simulink model "vr_octavia"  (Simulink 7.5)
settings: Solver=ode45  StartTime=0.0  StopTime=111.56  RelTol=1e-3
PostLoadFcn:
  | load octavia_testlap
libraries: vrlib x26, simulink x1
Description:
  | Vehicle Dynamics Visualization
  | 
  | The vr_octavia example shows the benefits of visualization of complex dynamic model
  | in the virtual reality environment. It also demonstrates Simulink(R) 3D Animation(TM)
  | 3D off-line animation recording functionality.
  | 
  | The pre-computed simulation data, representing one lap of a vehicle on a testing circuit,
  | is converted from dynamic model signal structure into the form that can be sent
  | to the virtual reality scene. This conversion includes splitting the combined signals
  | into signals governing individual VRML objects properties and coordinate systems
  | transformations. The data is then sent to the virtual reality scene using
  | VR Sink block with sample rate 25 Hz.
  | 
  | The dynamic model provides not only signals that influence visual properties of objects
  | (positions and rotations), but also forces and other similar quantities, that can be
  | visualized as well. In this example, wheel forces are visualized using VRML triads
  | scaled dynamically according to current force values. Force triads can be switched off
  | by the Forces Visibility Switch.
  | 
  | When working with virtual reality models, there is a common requirement to track
  | certain moving objects with the camera. Usually, the direction from the camera
  | to the object is easily available (both positions are known, so direction from
  | the camera to the object is defined as the difference between the two positions).
  | Because in VRML the viewpoint orientation is defined in the form of 4-element [axis angle]
  | VRML rotation, camera direction must be converted into this format before sending
  | to virtual scene. Simulink 3D Animation provides the Viewpoint Direction to VRML Orientation
  | block to perform this conversion. In this example, switch to the "Simulink Controlled Viewpoint"
  | in the viewer to see the camera tracking effect.
  | 
  | Simulink 3D Animation allows two methods of recording animation files - 2D animation (AVI files)
  | and 3D animation (VRML files). Here we describe how a 3D VRML animation file can be
  | created and further used. In the internal viewer Recording menu select the
  | Capture and Recording Parameters... option.
  | 
  | In the Capture and Recording Parameters dialog, select the Record to VRML checkbox.
  | Leave the File: editbox at its default value. Select the Scheduled Recording mode
  | and specify the time period for which you want to record the offline animation time.
  | Here we record the animation during the entire simulation time defined for this model,
  | you may select any time interval between the Simulink model Start time and Stop time.
  | For details on recording parameters please refer to the product documentation.
  | 
  | Once you define these animation recording parameters, animation file is created
  | automatically when you start the simulation. Unlike with creating the 2D animation files,
  | the internal viewer figure can be minimized during simulation, which significantly speeds up
  | the simulation. At the end of simulation run, the created VRML animation file
  | octavia_scene_anim_1.wrl remains in the working directory for later use.
  | 
  | If you distribute animation files, make sure to also distribute all the inlined object and texture
  | files referenced in the original VRML world file.
  | 
  | In the case of this demonstration example, the following files must be distributed together
  | with the resulting animation file octavia_scene_anim_1.wrl :
  | 
  |     * octavia_body.wrl
  |     * octavia_road.wrl
  |     * triad.wrl
  |     * /texture/octavia_*.jpg
  | 
  | As the VRML animation file is created by default into the current working directory,
  | and not the Simulink 3D Animation demos directory, you will need to copy all these
  | files to the current working directory to view the off-line animation file correctly.
  | 
  | Viewing VRML off-line animation file:
  | 
  | Let's assume that you want to view the octavia_scene_anim_1.wrl file that is in your
  | current working directory. You can play and inspect this animated file with comfort
  | using the VR Animation Player tool:
  | 
  |     vrplay('octavia_scene_anim_1.wrl');
  | 
  | You can view the resulting VRML animation file also using Orbisnap, blaxxun Contact
  | or any other generally available VRML97 viewer, or using Simulink 3D Animation
  | Internal Viewer. When using the internal viewer, it is necessary to set the virtual world
  | TimeSource property to freerun to be able to see the animation. Issue the following
  | commands at the MATLAB(R) command window:
  | 
  |     w=vrview('octavia_scene_anim_1.wrl');
  |     set(w, 'TimeSource', 'freerun');
  | 
  | A VRML animation file based on this example is pre-recorded in the /vrdemos directory
  | under the following name:
  | 
  |     octavia_scene_anim.wrl
  | 
  | Acknowledgements:
  | 
  | Skoda Octavia model copyright Skoda Auto, courtesy of Ismar VR, Czech Republic.
  | Road geometry and simulation data generated using veDYNA by TESIS DYNAware, Germany.
settings Model: Creator=Sehnal  LastModifiedBy=Danek  ExtModeArmWhenConnect=off  BufferReuse=off
settings DataIOCC: SignalLoggingName=sigsOut
settings OptimizationCC: BooleanDataType=off  InlineInvariantSignals=on  OptimizeBlockIOStorage=off  BufferReuse=off  ExpressionFolding=off  LocalBlockOutputs=off  InitFltsAndDblsToZero=on
settings DebuggingCC: CheckExecutionContextPreStartOutputMsg=on  CheckExecutionContextRuntimeOutputMsg=on  SignalResolutionControl=TryResolveAllWithWarning  SolverPrmCheckMsg=none  MultiTaskDSMMsg=warning  MultiTaskCondExecSysMsg=none  StrictBusMsg=None
settings RTWCC: RetainRTWFile=on  ProcessScript=grt_make_rtw_hook  IncludeERTFirstTime=on
settings GRTTargetCC: TargetFcnLib=ansi_tfl_tmw.mat

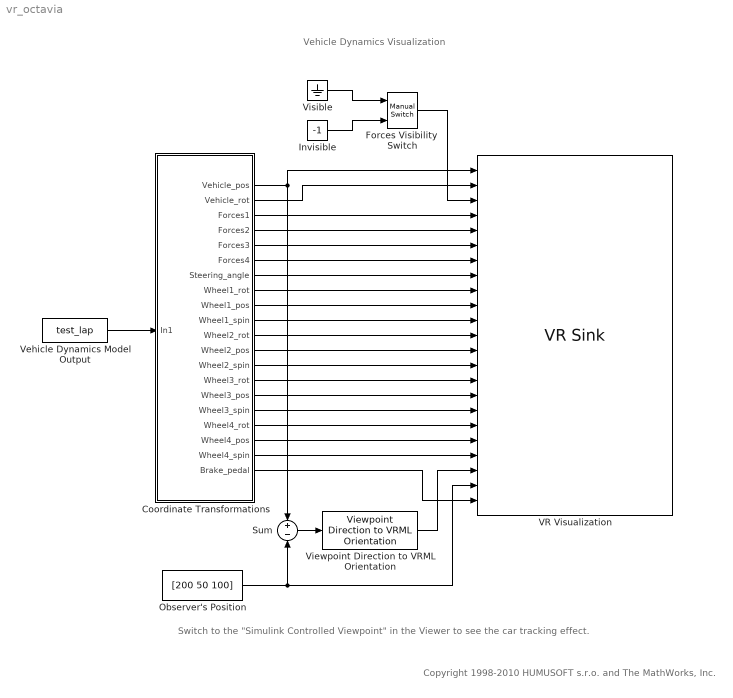
== system vr_octavia ==
  note: Vehicle Dynamics Visualization
  note: Switch to the "Simulink Controlled Viewpoint"
      | in the Viewer to see the car tracking effect.
  note: Copyright 1998-2010 HUMUSOFT s.r.o. and The MathWorks, Inc.
  Coordinate Transformations : Subsystem
  Forces Visibility  Switch : simulink/Signal Routing/Manual Switch  SystemSampleTime=-1  sw=1  action=0  varsize=off
  Invisible : Constant  Value=-1  OutDataType=sfix(16)  OutScaling=2^0
  Observer's Position : Constant  Value=[200 50 100]  OutDataType=sfix(16)  OutScaling=2^0
  Sum : Sum  Inputs=+-  OutDataType=sfix(16)  OutScaling=2^0
  VR Visualization : vrlib/VR Sink  InstantiateOnLoad=on  SampleTime=0.04  ViewEnable=on  RemoteChange=off  RemoteView=on  FieldsWritten=Vehicle_pos_Car1.translation.3.1.double#Vehicle_rot_Car1.rotation.4.1.double#Forces_visible_Car1.whichChoice.1.1.double#Force1_Car1.scale.3.1.double#Force2_Car1.scale.3.1.double#Force3_Car1.scale.3.1.double#Force4_Car1.scale.3.1.double#SteeringWheelAngle1_Car1.rotation.4.1.double#WheelFL_Car1.rotation.4.1.double#WheelFL_Car1.translation.3.1.double#WheelSpinFL_Car1.rotation.4.1.double#WheelFR_Car1.rotation.4.1.double#WheelFR_Car1.translation.3.1.double#WheelSpinFR_Car1.rotation.4.1.double#WheelRL_Car1.rotation.4.1.double#WheelRL_Car1.translation.3.1.double#WheelSpinRL_Car1.rotation.4.1.double#WheelRR_Car1.rotation.4.1.double#WheelRR_Car1.translation.3.1.double#WheelSpinRR_Car1.rotation.4.1.double#FlyingCamera.orientation.4.1.double#FlyingCamera.position.3.1.double#Brake_Switch_Car1.whichChoice.1.1.double  WorldFileName=octavia_scene.wrl  WorldDescription=Vehicle Dynamics Visualization - Skoda Octavia  AutoView=on  VideoDimensions=[]  FigureProperties="{'Position', 'Name', 'Viewpoint', 'CameraBound', 'CameraDirection', 'CameraPosition', 'CameraUpVector', 'ZoomFactor', 'Antialiasing', 'Headlight', 'Lighting', 'NavPanel', 'StatusBar', 'ToolBar', 'Textures', 'Transparency', 'Wireframe', 'NavZones', 'NavMode', 'NavSpeed', 'Record2DCompressMethod', 'Record2DCompressQuality', 'Record2D', 'Record2DFileName', 'Record2DFPS'; [1.3000000000000000e+001  7.7000000000000000e+001  5.7600000000000000e+002  3.8000000000000000e+002], 'Vehicle Dynamics Visualization - Skoda Octavia', 'Car - View from Right Above Ahead', 'on', [0.0000000000000000e+000  0.0000000000000000e+000 -1.0000000000000000e+000], [0.0000000000000000e+000  0.0000000000000000e+000  0.0000000000000000e+000], [0.0000000000000000e+000  1.0000000000000000e+000  0.0000000000000000e+000], [1.0000000000000000e+000], 'off', 'off', 'on', 'halfbar', 'off', 'on', 'on', 'on', 'off', 'off', 'walk', 'normal', 'auto', [7.5000000000000000e+001], 'off', '%f_anim_%n.avi', [1.5000000000000000e+001]}"
  Vehicle Dynamics Model Output : FromWorkspace  VariableName=test_lap  SampleTime=0.04  OutputAfterFinalValue=Holding final value
  Viewpoint Direction to VRML Orientation : vrlib/Utilities/Viewpoint Direction to VRML Orientation  SystemSampleTime=-1
  Visible : Ground
  wires:
  Visible/1 -> Forces Visibility  Switch/1
  Invisible/1 -> Forces Visibility  Switch/2
  Vehicle Dynamics Model Output/1 -> Coordinate Transformations/1(In1)
  Coordinate Transformations/1(Vehicle_pos) -> VR Visualization/1, Sum/1
  Coordinate Transformations/2(Vehicle_rot) -> VR Visualization/2
  Forces Visibility  Switch/1 -> VR Visualization/3
  Coordinate Transformations/3(Forces1) -> VR Visualization/4
  Coordinate Transformations/4(Forces2) -> VR Visualization/5
  Coordinate Transformations/5(Forces3) -> VR Visualization/6
  Coordinate Transformations/6(Forces4) -> VR Visualization/7
  Coordinate Transformations/7(Steering_angle) -> VR Visualization/8
  Coordinate Transformations/8(Wheel1_rot) -> VR Visualization/9
  Coordinate Transformations/9(Wheel1_pos) -> VR Visualization/10
  Coordinate Transformations/10(Wheel1_spin) -> VR Visualization/11
  Coordinate Transformations/11(Wheel2_rot) -> VR Visualization/12
  Coordinate Transformations/12(Wheel2_pos) -> VR Visualization/13
  Coordinate Transformations/13(Wheel2_spin) -> VR Visualization/14
  Coordinate Transformations/14(Wheel3_rot) -> VR Visualization/15
  Coordinate Transformations/15(Wheel3_pos) -> VR Visualization/16
  Coordinate Transformations/16(Wheel3_spin) -> VR Visualization/17
  Coordinate Transformations/17(Wheel4_rot) -> VR Visualization/18
  Coordinate Transformations/18(Wheel4_pos) -> VR Visualization/19
  Coordinate Transformations/19(Wheel4_spin) -> VR Visualization/20
  Coordinate Transformations/20(Brake_pedal) -> VR Visualization/23
  Sum/1 -> Viewpoint Direction to VRML Orientation/1
  Viewpoint Direction to VRML Orientation/1 -> VR Visualization/21
  Observer's Position/1 -> VR Visualization/22, Sum/2

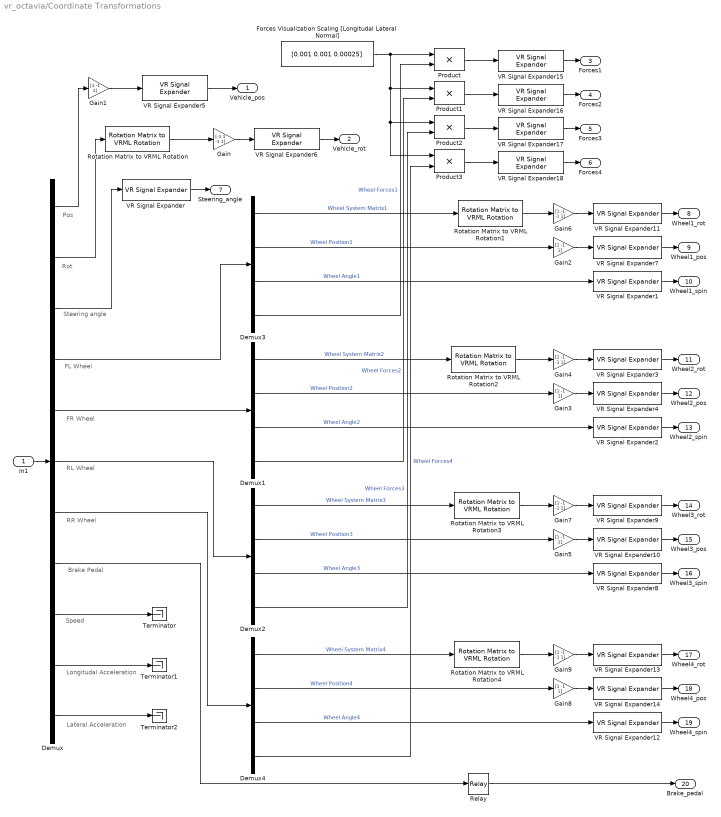
== system vr_octavia/Coordinate Transformations ==
  note: Steering angle
  note: FL Wheel
  note: FR Wheel
  note: RL Wheel
  note: RR Wheel
  note: Brake Pedal
  note: Pos
  note: Rot
  note: Speed
  note: Longitudal Acceleration
  note: Lateral Acceleration
  In1 : Inport  OutDataType=sfix(16)  OutScaling=2^0
  Demux : Demux  Outputs=[3,9,1,16,16,16,16,1,1,1,1]
  Demux{1..4} (4 alike) : Demux  Outputs=[9,3,1,3]
  Forces Visualization Scaling [Longitudal Lateral Normal] : Constant  Value=[0.001 0.001 0.00025]  OutDataType=sfix(16)  OutScaling=2^0
  Gain : Gain  Gain=[-1 1 -1 1]  ParameterDataType=sfix(16)  ParameterScaling=2^0  OutDataType=sfix(16)  OutScaling=2^0  SaturateOnIntegerOverflow=on  OutDataTypeStr=Inherit: Same as input  ParamDataTypeStr=Inherit: Same as input
  Gain{1..3,5,8} (5 alike) : Gain  Gain=[1 -1 1]  ParameterDataType=sfix(16)  ParameterScaling=2^0  OutDataType=sfix(16)  OutScaling=2^0  SaturateOnIntegerOverflow=on  OutDataTypeStr=Inherit: Same as input  ParamDataTypeStr=Inherit: Same as input
  Gain{4,6..7,9} (4 alike) : Gain  Gain=[1 -1 -1 1]  ParameterDataType=sfix(16)  ParameterScaling=2^0  OutDataType=sfix(16)  OutScaling=2^0  SaturateOnIntegerOverflow=on  OutDataTypeStr=Inherit: Same as input  ParamDataTypeStr=Inherit: Same as input
  Product{,1..3} (4 alike) : Product  OutDataType=sfix(16)  OutScaling=2^0  SaturateOnIntegerOverflow=on  OutDataTypeStr=Inherit: Same as first input
  Relay : Relay  OutDataType=sfix(16)  OutScaling=2^0
  Rotation Matrix to VRML Rotation{,1..4} (5 alike) : vrlib/Utilities/Rotation Matrix to VRML Rotation  SystemSampleTime=-1  maxzero=1e-12
  Terminator : Terminator
  Terminator1 : Terminator
  Terminator2 : Terminator
  VR Signal Expander{,1..2,8,12} (5 alike) : vrlib/VR Signal Expander  SystemSampleTime=-1  outwidth=4  outidx=[4]
  VR Signal Expander{4,7,10,14} (4 alike) : vrlib/VR Signal Expander  SystemSampleTime=-1  outwidth=3  outidx=[1 3 2 ]
  VR Signal Expander{3,6,9,11,13} (5 alike) : vrlib/VR Signal Expander  SystemSampleTime=-1  outwidth=4  outidx=[1 3 2 4]
  VR Signal Expander{5,15..18} (5 alike) : vrlib/VR Signal Expander  SystemSampleTime=-1  outwidth=3  outidx=[1 3 2]
  Vehicle_pos : Outport  OutDataType=sfix(16)  OutScaling=2^0
  Vehicle_rot : Outport  Port=2  OutDataType=sfix(16)  OutScaling=2^0
  Forces1 : Outport  Port=3  OutDataType=sfix(16)  OutScaling=2^0
  Forces2 : Outport  Port=4  OutDataType=sfix(16)  OutScaling=2^0
  Forces3 : Outport  Port=5  OutDataType=sfix(16)  OutScaling=2^0
  Forces4 : Outport  Port=6  OutDataType=sfix(16)  OutScaling=2^0
  Steering_angle : Outport  Port=7  OutDataType=sfix(16)  OutScaling=2^0
  Wheel1_rot : Outport  Port=8  OutDataType=sfix(16)  OutScaling=2^0
  Wheel1_pos : Outport  Port=9  OutDataType=sfix(16)  OutScaling=2^0
  Wheel1_spin : Outport  Port=10  OutDataType=sfix(16)  OutScaling=2^0
  Wheel2_rot : Outport  Port=11  OutDataType=sfix(16)  OutScaling=2^0
  Wheel2_pos : Outport  Port=12  OutDataType=sfix(16)  OutScaling=2^0
  Wheel2_spin : Outport  Port=13  OutDataType=sfix(16)  OutScaling=2^0
  Wheel3_rot : Outport  Port=14  OutDataType=sfix(16)  OutScaling=2^0
  Wheel3_pos : Outport  Port=15  OutDataType=sfix(16)  OutScaling=2^0
  Wheel3_spin : Outport  Port=16  OutDataType=sfix(16)  OutScaling=2^0
  Wheel4_rot : Outport  Port=17  OutDataType=sfix(16)  OutScaling=2^0
  Wheel4_pos : Outport  Port=18  OutDataType=sfix(16)  OutScaling=2^0
  Wheel4_spin : Outport  Port=19  OutDataType=sfix(16)  OutScaling=2^0
  Brake_pedal : Outport  Port=20  OutDataType=sfix(16)  OutScaling=2^0
  wires:
  Gain1/1 -> VR Signal Expander5/1
  Rotation Matrix to VRML Rotation/1 -> Gain/1
  Gain/1 -> VR Signal Expander6/1
  Gain6/1 -> VR Signal Expander11/1
  Gain2/1 -> VR Signal Expander7/1
  Demux3/1 -> Rotation Matrix to VRML Rotation1/1  "Wheel System Matrix1"
  Demux3/2 -> Gain2/1  "Wheel Position1"
  Demux3/3 -> VR Signal Expander1/1  "Wheel Angle1"
  Gain4/1 -> VR Signal Expander3/1
  Rotation Matrix to VRML Rotation2/1 -> Gain4/1
  Gain3/1 -> VR Signal Expander4/1
  Demux1/1 -> Rotation Matrix to VRML Rotation2/1  "Wheel System Matrix2"
  Demux1/2 -> Gain3/1  "Wheel Position2"
  Demux1/3 -> VR Signal Expander2/1  "Wheel Angle2"
  Gain7/1 -> VR Signal Expander9/1
  Rotation Matrix to VRML Rotation3/1 -> Gain7/1
  Demux2/4 -> Product2/2  "Wheel Forces3"
  Gain5/1 -> VR Signal Expander10/1
  Demux2/1 -> Rotation Matrix to VRML Rotation3/1  "Wheel System Matrix3"
  Demux2/2 -> Gain5/1  "Wheel Position3"
  Demux2/3 -> VR Signal Expander8/1  "Wheel Angle3"
  Gain9/1 -> VR Signal Expander13/1
  Rotation Matrix to VRML Rotation4/1 -> Gain9/1
  Demux4/4 -> Product3/2  "Wheel Forces4"
  Gain8/1 -> VR Signal Expander14/1
  Demux4/1 -> Rotation Matrix to VRML Rotation4/1  "Wheel System Matrix4"
  Demux4/2 -> Gain8/1  "Wheel Position4"
  Demux4/3 -> VR Signal Expander12/1  "Wheel Angle4"
  VR Signal Expander5/1 -> Vehicle_pos/1
  Demux3/4 -> Product/2  "Wheel Forces1"
  Demux1/4 -> Product1/2  "Wheel Forces2"
  Product/1 -> VR Signal Expander15/1
  Product1/1 -> VR Signal Expander16/1
  Product2/1 -> VR Signal Expander17/1
  Product3/1 -> VR Signal Expander18/1
  VR Signal Expander6/1 -> Vehicle_rot/1
  VR Signal Expander15/1 -> Forces1/1
  VR Signal Expander16/1 -> Forces2/1
  VR Signal Expander17/1 -> Forces3/1
  VR Signal Expander18/1 -> Forces4/1
  VR Signal Expander/1 -> Steering_angle/1
  VR Signal Expander11/1 -> Wheel1_rot/1
  In1/1 -> Demux/1
  VR Signal Expander7/1 -> Wheel1_pos/1
  VR Signal Expander1/1 -> Wheel1_spin/1
  VR Signal Expander3/1 -> Wheel2_rot/1
  VR Signal Expander4/1 -> Wheel2_pos/1
  VR Signal Expander2/1 -> Wheel2_spin/1
  VR Signal Expander9/1 -> Wheel3_rot/1
  VR Signal Expander10/1 -> Wheel3_pos/1
  VR Signal Expander8/1 -> Wheel3_spin/1
  VR Signal Expander13/1 -> Wheel4_rot/1
  VR Signal Expander14/1 -> Wheel4_pos/1
  VR Signal Expander12/1 -> Wheel4_spin/1
  Demux/8 -> Relay/1
  Relay/1 -> Brake_pedal/1
  Demux/1 -> Gain1/1
  Demux/2 -> Rotation Matrix to VRML Rotation/1
  Demux/3 -> VR Signal Expander/1
  Demux/4 -> Demux3/1
  Demux/5 -> Demux1/1
  Demux/6 -> Demux2/1
  Demux/7 -> Demux4/1
  Forces Visualization Scaling [Longitudal Lateral Normal]/1 -> Product/1, Product1/1, Product2/1, Product3/1
  Rotation Matrix to VRML Rotation1/1 -> Gain6/1
  Demux/9 -> Terminator/1
  Demux/10 -> Terminator1/1
  Demux/11 -> Terminator2/1
